simulink model "Question8no"  (R2020a)
settings: Solver=VariableStepAuto  StartTime=0.0  StopTime=10.0  RelTol=1e-3
libraries: simulink x2
settings Model: Creator=anjal  LastModifiedBy=anjal

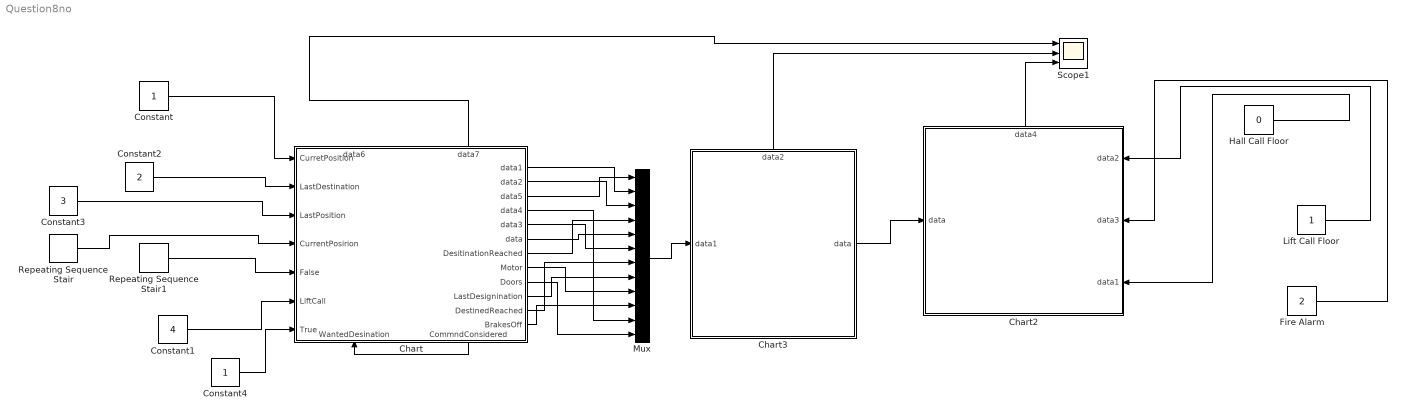
== system Question8no ==
  Chart : Stateflow chart  TreatAsAtomicUnit=on
      settings: PortSchema="{\"entries\":[{\"content\":{\"sides\":[{\"content\":{\"connectorIds\":[\"In1\",\"In2\",\"In3\",\"In4\",\"In5\",\"In6\",\"In7\"]},\"type\":\"ConnectorPlacement.EquallySpacedRectSide\",\"uuid\":\"aa2a2372-4a10-4770-bff8-2a5b90af5b20\"},{\"content\":{\"connectorIds\":[\"Out3\",\"Out4\",\"Out5\",\"Out6\",\"Out7\",\"Out8\",\"Out9\",\"Out10\",\"Out11\",\"Out12\",\"Out13\",\"Out14\"],\"side\":\"RIGHT\"},\"type\":\"ConnectorPlacement.EquallySpacedRectSide\",\"uuid\":\"a7af34cf-c437-4d78-8acf-45216a4d139b\"},{\"content\":{\"connectorIds\":[\"Out1\",\"Out2\"],\"side\":\"TOP\"},\"type\":\"ConnectorPlacement.EquallySpacedRectSide\",\"uuid\":\"3bd3ce64-d1bb-42fd-9d27-36936f7a2810\"},{\"content\":{\"connectorIds\":[\"In8\",\"Out15\"],\"side\":\"BOTTOM\"},\"type\":\"ConnectorPlacement.EquallySpacedRectSide\",\"uuid\":\"d2813dea-9bc2-4483-a724-644ca05e2280\"}]},\"type\":\"ConnectorPlacement.EquallySpacedConnector\",\"uuid\":\"2220a9f5-bcd6-4180-bb9f-0eefc9aaef0c\"}],\"packageUris\":[\"http://schema.mathworks.com/mf0/Connector/19700101\"],\"version\":\"1.0\"}"
  Chart2 : Stateflow chart  TreatAsAtomicUnit=on
      settings: PortSchema="{\"entries\":[{\"content\":{\"sides\":[{\"content\":{\"connectorIds\":[\"In4\"]},\"type\":\"ConnectorPlacement.EquallySpacedRectSide\",\"uuid\":\"9d12e941-f93e-4b81-ba54-9a45c14cbce8\"},{\"content\":{\"connectorIds\":[\"In1\",\"In2\",\"In3\"],\"side\":\"RIGHT\"},\"type\":\"ConnectorPlacement.EquallySpacedRectSide\",\"uuid\":\"45bb56a4-cc23-4366-923d-37100c39de85\"},{\"content\":{\"connectorIds\":[\"Out1\"],\"side\":\"TOP\"},\"type\":\"ConnectorPlacement.EquallySpacedRectSide\",\"uuid\":\"f9aae596-f753-4979-aba1-1b0e4382f01c\"}]},\"type\":\"ConnectorPlacement.EquallySpacedConnector\",\"uuid\":\"93073253-c852-46b5-9272-3cf50cfecfd7\"}],\"packageUris\":[\"http://schema.mathworks.com/mf0/Connector/19700101\"],\"version\":\"1.0\"}"
  Chart3 : Stateflow chart  TreatAsAtomicUnit=on
      settings: PortSchema="{\"entries\":[{\"content\":{\"sides\":[{\"content\":{\"connectorIds\":[\"In1\"]},\"type\":\"ConnectorPlacement.EquallySpacedRectSide\",\"uuid\":\"d9b4708a-5ec2-415c-9bcb-1c90d346baa5\"},{\"content\":{\"connectorIds\":[\"Out2\"],\"side\":\"RIGHT\"},\"type\":\"ConnectorPlacement.EquallySpacedRectSide\",\"uuid\":\"f3e2e2d4-e6bf-4a2d-9fb3-4788f59b00ae\"},{\"content\":{\"connectorIds\":[\"Out1\"],\"side\":\"TOP\"},\"type\":\"ConnectorPlacement.EquallySpacedRectSide\",\"uuid\":\"1f665c11-962c-408c-96a7-5a8b252d7ed4\"}]},\"type\":\"ConnectorPlacement.EquallySpacedConnector\",\"uuid\":\"6839c0ad-ebd9-4c9c-9eba-b3c377919bad\"}],\"packageUris\":[\"http://schema.mathworks.com/mf0/Connector/19700101\"],\"version\":\"1.0\"}"
  Constant : Constant
  Constant1 : Constant  Value=4
  Constant2 : Constant  Value=2
  Constant3 : Constant  Value=3
  Constant4 : Constant
  Fire Alarm : Constant  Value=2
  Hall Call Floor : Constant  Value=0
  Lift Call Floor : Constant
  Mux : Mux  Inputs=12
  Repeating Sequence Stair : simulink/Sources/Repeating Sequence Stair  OutValues=[3 1 4 2 1].'  tsamp=-1  OutMin=[]  OutMax=[]  OutDataTypeStr=double  OutputDataTypeScalingMode=double  OutDataType=fixdt(0,8)  ConRadixGroup=Best Precision: Vector-wise  OutScaling=2^-12
  Repeating Sequence Stair1 : simulink/Sources/Repeating Sequence Stair  OutValues=[3 1 4 2 1].'  tsamp=-1  OutMin=[]  OutMax=[]  OutDataTypeStr=double  OutputDataTypeScalingMode=double  OutDataType=fixdt(0,8)  ConRadixGroup=Best Precision: Vector-wise  OutScaling=2^-12
  Scope1 : Scope  NumInputPorts=3
  wires:
  Constant4/1 -> Chart/7(True)
  Constant3/1 -> Chart/3(LastPosition)
  Chart/10(Motor) -> Mux/9
  Repeating Sequence Stair1/1 -> Chart/5(False)
  Chart/14(BrakesOff) -> Mux/10
  Chart/9(DesitinationReached) -> Mux/4
  Chart/13(DestinedReached) -> Mux/7
  Chart/15(CommndConsidered) -> Chart/8(WantedDesination)
  Chart2/1(data4) -> Scope1/3
  Chart/2(data7) -> Scope1/1
  Chart3/1(data2) -> Scope1/2
  Mux/1 -> Chart3/1(data1)
  Lift Call Floor/1 -> Chart2/1(data2)
  Chart3/2(data) -> Chart2/4(data)
  Fire Alarm/1 -> Chart2/2(data3)
  Chart/4(data2) -> Mux/3
  Chart/6(data4) -> Mux/11
  Hall Call Floor/1 -> Chart2/3(data1)
  Chart/5(data5) -> Mux/1
  Chart/7(data3) -> Mux/6
  Repeating Sequence Stair/1 -> Chart/4(CurrentPosirion)
  Constant2/1 -> Chart/2(LastDestination)
  Constant1/1 -> Chart/6(LiftCall)
  Constant/1 -> Chart/1(CurretPosition)
  Chart/11(Doors) -> Mux/12
  Chart/3(data1) -> Mux/2
  Chart/12(LastDesignination) -> Mux/8
  Chart/8(data) -> Mux/5

== stateflow chart Question8no/Chart ==
  state Stopped
    state Stopped_and_Waiting
      state Initializing
        entry:Motor=false;BrakesOff=false;Doors=false;
        DestinedReached=False;CommndConsidered=false;
      state FixingDesignation
        LastDesignination=WantedDesination;
      state SettingDown
        entry:Up=false;
      state SettingUp
        entry:Up=true
      state CommandAccepted
        CommandConsidered=true;
      (default) -> Initializing [order 1] : [LiftCall&&~CommandConsidered]
      Initializing -> FixingDesignation
      FixingDesignation -> SettingDown [order 3]
      FixingDesignation -> SettingUp [order 1] : [CurretPosition<LastPosition]
      (default) -> CommandAccepted [order 2]
    state Stopping_at_destination
      state StoppingLift
        entry:Motor=False;BrakesOff=False;
      state ErrorState
        entry:Doors=false;
      state OpeningDoors
        entry:DesitinationReached=True;Doors=true;
      (default) -> StoppingLift
      StoppingLift -> OpeningDoors [order 1] : [CurrentPosition~=LastDestination]
      StoppingLift -> ErrorState [order 2]
    (default) -> Stopped_and_Waiting
    FixingDesignation -> Stopping_at_destination [order 2] : [CurrentPosition==LastDestination]
  state Moving
    state StartingMotor
      entry:Motor=true;BrakesOff=true;Doors=false;
    state MovingUp
      entry:CurrentPosition=CurrentPosition + 1
    state MovingDown
      entry:CurrentPosition = CurrentPosition-1;
    (default) -> StartingMotor
    MovingDown -> MovingDown : [CurrentPosirion>LastDestination]
    MovingUp -> MovingUp : [CurrentPosition<LastDestination]
    StartingMotor -> MovingUp [order 1] : [Up]
    StartingMotor -> MovingDown [order 2] : [~Up]
  (default) -> Stopped
  Moving -> Stopping_at_destination : [CurrentPosition==LastPosition]
  Stopped_and_Waiting -> Moving : [CommandConsidered]
  data: data6 output; data7 output; data1 output; data2 output; data5 output; data4 output; data3 output; data output; CurretPosition input; LastDestination input; LastPosition input; CurrentPosirion input; False input; LiftCall input; True input; WantedDesination input; DesitinationReached output; Motor output; Doors output; LastDesignination output; DestinedReached output; BrakesOff output; CommndConsidered output; CurrentPosition local; Up local; CommandConsidered local

== stateflow chart Question8no/Chart3 ==
  state Elevator
    state Indside_Elevator_A
      state Off
        entry:
        Lift=0;
        state noSwitch
        state carSwitch
        (default) -> Elevator.Indside_Elevator_A.Off.noSwitch
        Elevator.Indside_Elevator_A.Off.noSwitch -> Elevator.Indside_Elevator_A.Off.carSwitch : [after(3,tick)]
      state carOn
        entry:
        lift=1;
      state liftoff
        entry:
        lift=-1;
      (default) -> Off
      carOn -> Off : [car2 > (car3-dT)]
      liftoff -> Off : [car2< (car3+dT)]
      Elevator.Indside_Elevator_A.Off.carSwitch -> carOn [order 1] : [car < (car-dT)]
      Elevator.Indside_Elevator_A.Off.carSwitch -> liftoff [order 2] : [car > (car+dT)]
    state ElevatorOff
      entry:
      LiftEntry=0;
      state noSwitch
      state carSwitch
      (default) -> Elevator.ElevatorOff.noSwitch
      Elevator.ElevatorOff.noSwitch -> Elevator.ElevatorOff.carSwitch : [after(3,tick)]
    (default) -> Indside_Elevator_A
    Indside_Elevator_A -> ElevatorOff : [car == 0]
    Elevator.ElevatorOff.carSwitch -> Indside_Elevator_A : [car == 1]
  data: data2 output; data output; data1 input

== stateflow chart Question8no/Chart2 ==
  state LiftControl1
    du: updateLiftcontrol;
    state Normal
    state Upshift
      en: count = 0;
      du: count = count+1;
    state Downshift
      en: count = 0;
      du: count = count+1;
    (default) -> Normal
    Normal -> Upshift [order 1] : [v>v_liftup]
        | /{Lift.UP;}
    Normal -> Downshift [order 2] : [v<v_liftdown]
        | /{Lift.DOWN;}
    Downshift -> Normal : [count > 3]
    Upshift -> Normal : [count > 3]
  state LiftControl
    state Floor_2
      en: floor= 2;
    state Floor_4
      en: floor = 4;
    state Floor_5
      en: floor = 4;
    state Floor_3
      en: floor = 3;
    state Floor_1
      en: floor = 1;
    (default) -> Floor_1
    Floor_2 -> Floor_3 [order 1] : UP
    Floor_1 -> Floor_2 : UP
    Floor_3 -> Floor_4 [order 1] : UP
    Floor_4 -> Floor_5 [order 2]
    Floor_5 -> Floor_4
    Floor_2 -> Floor_1 [order 2] : DOWN
    Floor_3 -> Floor_2 [order 2] : DOWN
    Floor_4 -> Floor_3 [order 1] : DOWN
  (default) -> LiftControl1 [order 1] : Liftcall
  (default) -> LiftControl [order 2]
  data: data2 input; data3 input; data1 input; data input; data4 output
  events: UP local FUNCTION_CALL_EVENT; DOWN local FUNCTION_CALL_EVENT
